simulink model "doc_design_iteration_turbo"  (R2014a)
settings: Solver=VariableStepDiscrete  StartTime=0.0  StopTime=inf  RelTol=1e-3
PreLoadFcn:
  | EbNo=0;
  | maxNumErrs=200;
  | maxNumBits=1e8;
  | load Parameters.mat
libraries: commdigbbndpm3 x2, commcnvcod2 x2, commchan3 x1, commrandsrc2 x1, commsink2 x1
settings Model: Creator=The MathWorks Inc.
settings OptimizationCC: ExpressionDepthLimit=2147483647
settings DebuggingCC: UnderspecifiedInitializationDetection=Classic  StateNameClashWarn=warning
settings GRTTargetCC: CombineOutputUpdateFcns=off  GRTInterface=on

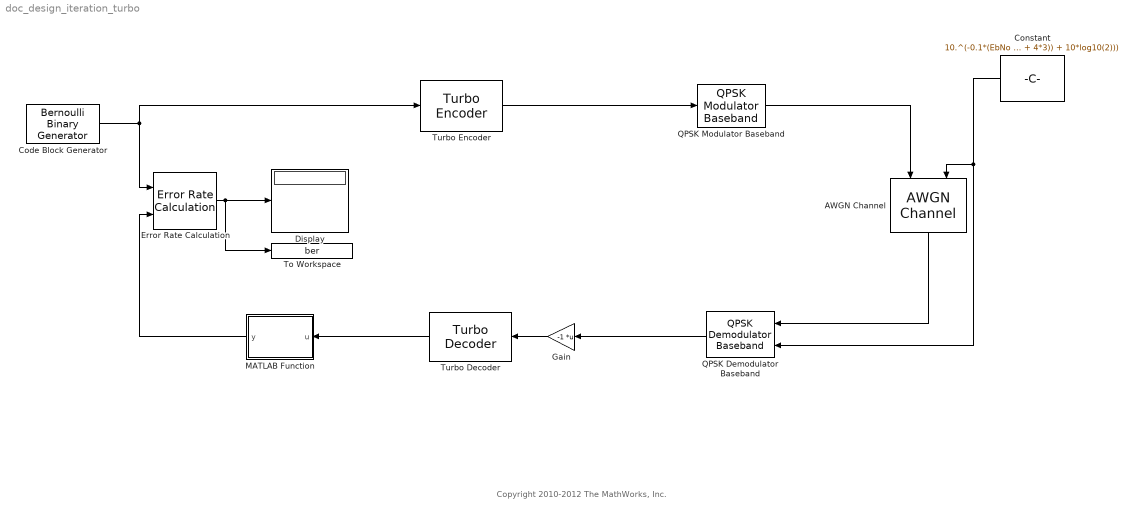
== system doc_design_iteration_turbo ==
  note: Copyright 2010-2012 The MathWorks, Inc.
  AWGN Channel : commchan3/AWGN Channel  InputProcessing=Columns as channels (frame based)  seed=67890  noiseMode=Variance from port  EbNodB=10  EsNodB=10  SNRdB=10  bitsPerSym=2  Ps=1  Tsym=1  variance=10.^(-0.1*(EbNo + 10*log10(1/2) + 10*log10(2)))
  Code Block Generator : commrandsrc2/Bernoulli Binary Generator  P=0.5  seed=12345  Ts=1/2048  frameBased=on  sampPerFrame=2048  orient=off  outDataType=double
  Constant : Constant  Value=10.^(-0.1*(EbNo + 10*log10(2048/(3*2048 + 4*3)) + 10*log10(2)))  VectorParams1D=off
  Display : Display
  Error Rate Calculation : commsink2/Error Rate Calculation  N=0  st_delay=0  cp_mode=Entire frame  subframe=[]  PMode=Port  WsName=ErrorVec1  RsMode2=off  stop=on  numErr=maxNumErrs  maxBits=maxNumBits
  Gain : Gain  Gain=-1  Multiplication=Matrix(K*u)
  MATLAB Function : MATLAB Function  TreatAsAtomicUnit=on
  QPSK Demodulator Baseband : commdigbbndpm3/QPSK Demodulator Baseband  Ph=0  Dec=Gray  OutType=Bit  DecType=Log-likelihood ratio  VarSource=Port  Variance=1  outDtype1=boolean  outDtype2=Inherit via internal rule  derotateFactorWordLen=16
  QPSK Modulator Baseband : commdigbbndpm3/QPSK Modulator Baseband  InType=Bit  Enc=Gray  Ph=0  outDtype=double  outWordLen=16  outUDDataType=sfix(16)  outFracLenMode=Best precision  outFracLen=15
  To Workspace : ToWorkspace  VariableName=ber  SampleTime=-1
      settings: MaxDataPoints=1
  Turbo Decoder : commcnvcod2/Turbo Decoder  SimulateUsing=Interpreted execution  TrellisStructure=poly2trellis(4, [13 15], 13)  InterleaverIndicesSource=Property  InterleaverIndices=turbo_interleaver  Algorithm=True APP  NumScalingBits=3  NumIterations=6
  Turbo Encoder : commcnvcod2/Turbo Encoder  SimulateUsing=Interpreted execution  TrellisStructure=poly2trellis(4, [13 15], 13)  InterleaverIndicesSource=Property  InterleaverIndices=turbo_interleaver
  wires:
  Code Block Generator/1 -> Turbo Encoder/1, Error Rate Calculation/1
  AWGN Channel/1 -> QPSK Demodulator Baseband/1
  Error Rate Calculation/1 -> Display/1, To Workspace/1
  QPSK Modulator Baseband/1 -> AWGN Channel/1
  Turbo Encoder/1 -> QPSK Modulator Baseband/1
  MATLAB Function/1(y) -> Error Rate Calculation/2
  Constant/1 -> QPSK Demodulator Baseband/2, AWGN Channel/2
  QPSK Demodulator Baseband/1 -> Gain/1
  Gain/1 -> Turbo Decoder/1
  Turbo Decoder/1 -> MATLAB Function/1(u)

== matlab function doc_design_iteration_turbo/MATLAB Function ==
  data: u input; y output
function y = fcn(u)
%#codegen

y = u(1:2048);
